simulink model "qusetion1_2"  (R2016b)
settings: Solver=VariableStepAuto  StartTime=0.0  StopTime=20  RelTol=1e-3
settings Model: Creator=dell  LastModifiedBy=dell
settings OptimizationCC: BooleanDataType=off

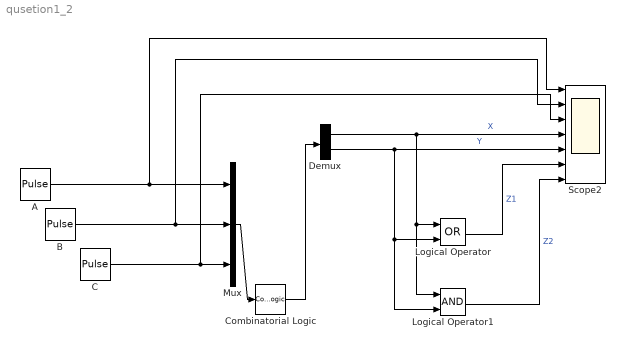
== system qusetion1_2 ==
  A : DiscretePulseGenerator  Period=8  PulseWidth=4
  B : DiscretePulseGenerator  Period=8  PulseWidth=4  PhaseDelay=1
  C : DiscretePulseGenerator  Period=8  PulseWidth=4  PhaseDelay=2
  Combinatorial Logic : CombinatorialLogic  TruthTable=[1 1;1 0;1 0;1 0;1 0;1 0;1 0;0 1]
  Demux : Demux  Outputs=2
  Logical Operator : Logic  Operator=OR  AllPortsSameDT=off  OutDataTypeStr=boolean
  Logical Operator1 : Logic  AllPortsSameDT=off  OutDataTypeStr=boolean
  Mux : Mux  Inputs=3
  Scope2 : Scope  NumInputPorts=7
  wires:
  A/1 -> Scope2/1, Mux/1
  B/1 -> Scope2/2, Mux/2
  C/1 -> Scope2/3, Mux/3
  Mux/1 -> Combinatorial Logic/1
  Combinatorial Logic/1 -> Demux/1
  Demux/2 -> Logical Operator1/2, Logical Operator/2, Scope2/5  "Y"
  Logical Operator1/1 -> Scope2/7  "Z2"
  Logical Operator/1 -> Scope2/6  "Z1"
  Demux/1 -> Scope2/4, Logical Operator1/1, Logical Operator/1  "X"
